simulink model "s_maglev_pid"  (R2021a)
settings: Solver=ode4  StartTime=0.0  StopTime=10.0  FixedStep=0.001  RelTol=1e-3
values from neighbouring files (symbols this model uses):
  g = 9.81    [config_maglev.m]
  IC_MAX = 3    [config_maglev.m]
  Kff_b = ic0 / xb0    [d_maglev_pi_piv.m]
  Ki_c = wn_c^2 * tau_c / Kc_dc    [d_maglev_pi_piv.m]
  Km = 6.5308e-5    (= 6.5308e-05)    [config_maglev.m]
  Kp_c = (2*zeta_c*wn_c*tau_c - 1) / Kc_dc    [d_maglev_pi_piv.m]
  Lc = 0.4125    [config_maglev.m]    (also in setup_maglev.m = 0.374)
  maglev_km = [xbfit; Km_xb_array]'    [load_variable_km.m]
  MAX_XB_WDUP = 1    [setup_maglev.m]
  Mb = 0.068    [config_maglev.m]
  Rc = 10    [config_maglev.m]    (also in setup_maglev.m)
  Tb = 0.014    [config_maglev.m]
  VMAX_AMP = 24    [config_maglev.m]
  xb0 = 6e-3    (= 0.006)    [setup_maglev.m]
  XB_REF_RATE = 5e-3    (= 0.005)    [setup_maglev.m]
undefined symbols (not defined in the file or in its folder): Ctuned, CtunedNom
libraries: pid_lib x2
settings Model: Creator=MLevis  LastModifiedBy=MLevis
settings DataIOCC: ReturnWorkspaceOutputs=off

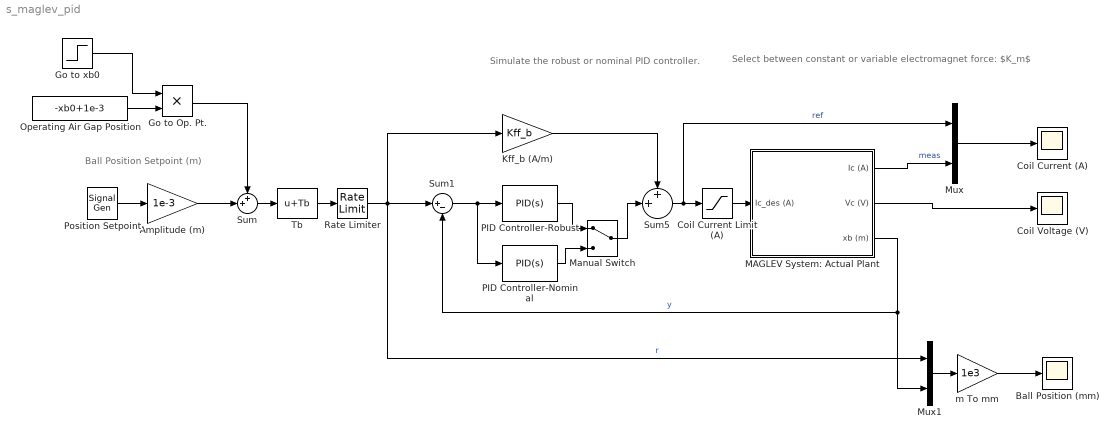
== system s_maglev_pid ==
  note: Simulate the robust or nominal PID controller.
  note: Select between constant or variable electromagnet force: $K_m$
  note: Ball Position Setpoint (m)
  Amplitude (m) : Gain  Gain=1e-3  SaturateOnIntegerOverflow=on  OutDataTypeStr=Inherit: Same as input  ParamDataTypeStr=Inherit: Same as input
  Ball Position (mm) : Scope
  Coil Current Limit (A) : Saturate  UpperLimit=IC_MAX  LowerLimit=0
  Coil Current (A) : Scope
  Coil Voltage (V) : Scope
  Go to Op. Pt. : Product  RndMeth=Zero
  Go to xb0 : Step  Time=2  SampleTime=0
  Kff_b (A/m) : Gain  Gain=Kff_b  SaturateOnIntegerOverflow=on  OutDataTypeStr=Inherit: Same as input  ParamDataTypeStr=Inherit: Same as input
  MAGLEV System: Actual Plant : Subsystem
  Manual Switch : ManualSwitch
  Mux : Mux  Inputs=2
  Mux1 : Mux  Inputs=2
  Operating Air Gap Position : Constant  Value=-xb0+1e-3
  PID Controller-Nominal : pid_lib/PID Controller  Controller=PID  Form=Parallel  TimeDomain=Continuous-time  UseExternalTs=off  SampleTime=-1  IntegratorMethod=Forward Euler  FilterMethod=Forward Euler  ControllerParametersSource=internal  P=CtunedNom.Kp  I=CtunedNom.Ki  D=CtunedNom.Kd  UseFilter=on  N=1/CtunedNom.Tf  TunerSelectOption=Transfer Function Based (PID Tuner App)  InitialConditionSource=internal  InitialConditionForIntegrator=0  InitialConditionForFilter=0  DifferentiatorICPrevScaledInput=0  ExternalReset=none  TrackingMode=off  Kt=1  LimitOutput=on  SatLimitsSource=internal  UpperSaturationLimit=MAX_XB_WDUP  LowerSaturationLimit=-MAX_XB_WDUP  LinearizeAsGain=on  AntiWindupMode=back-calculation  Kb=1  POutMin=[]  POutMax=[]  IOutMin=[]  IOutMax=[]  DOutMin=[]  DOutMax=[]  NOutMin=[]  NOutMax=[]  SumOutMin=[]  SumOutMax=[]  SaturationOutMin=[]  SaturationOutMax=[]  PParamMin=[]  PParamMax=[]  IParamMin=[]  IParamMax=[]  DParamMin=[]  DParamMax=[]  NParamMin=[]  NParamMax=[]  KbParamMin=[]  KbParamMax=[]  KtParamMin=[]  KtParamMax=[]  KbOutMin=[]  KbOutMax=[]  KtOutMin=[]  KtOutMax=[]  IntegratorOutMin=[]  IntegratorOutMax=[]  FilterOutMin=[]  FilterOutMax=[]  SumI1OutMin=[]  SumI1OutMax=[]  SumI2OutMin=[]  SumI2OutMax=[]  SumI3OutMin=[]  SumI3OutMax=[]  SumI4OutMin=[]  SumI4OutMax=[]  SumDOutMin=[]  SumDOutMax=[]  DifferentiatorOutMin=[]  DifferentiatorOutMax=[]  FilterDiffOutCoefMin=[]  FilterDiffOutCoefMax=[]  ReciprocalOutMin=[]  ReciprocalOutMax=[]  SumDenOutMin=[]  SumDenOutMax=[]  SumNumOutMin=[]  SumNumOutMax=[]  DivideOutMin=[]  DivideOutMax=[]  UdiffTsProdOutMin=[]  UdiffTsProdOutMax=[]  NTsProdOutMin=[]  NTsProdOutMax=[]  UintegralTsProdOutMin=[]  UintegralTsProdOutMax=[]  UngainTsProdOutMin=[]  UngainTsProdOutMax=[]  IntegratorContinuousStateAttributes=''  IntegratorStateMustResolveToSignalObject=off  IntegratorRTWStateStorageClass=Auto  FilterContinuousStateAttributes=''  FilterStateMustResolveToSignalObject=off  FilterRTWStateStorageClass=Auto  ParallelPVariant=InternalParameters  IdealPVariant=Disabled  IVariant=InternalParameters  DVariant=InternalParameters  IntegratorVariant=Continuous  SatVariant=Enabled  AWVariant=BackCalculation  PCopyVariant=Disabled  TRVariant=Disabled  FdbkBlocksVariant=Forward  IdealPFdbkVariant=Disabled  SatFdbkVariant=Disabled  DerivativeFilterVariant=ContFilter  NVariant=InternalParameters  NCopyVariant=Disabled  FilterICVariant=InternalICsFilter  IntegratorICVariant=InternalICs  ExternalResetVariant=Disabled  TRSumVariant=Passthrough  SumFdbkVariant=Disabled  SumVariant=Sum_PID  TsampFilterVariant=InternalTs  TsampNgainVariant=Passthrough  TsampIntegralVariant=Passthrough  ExternalSaturationOutDataTypeStr=Inherit: Same as second input
  PID Controller-Robust : pid_lib/PID Controller  Controller=PID  Form=Parallel  TimeDomain=Continuous-time  UseExternalTs=off  SampleTime=-1  IntegratorMethod=Forward Euler  FilterMethod=Forward Euler  ControllerParametersSource=internal  P=Ctuned.Kp  I=Ctuned.Ki  D=Ctuned.Kd  UseFilter=on  N=1/Ctuned.Tf  TunerSelectOption=Transfer Function Based (PID Tuner App)  InitialConditionSource=internal  InitialConditionForIntegrator=0  InitialConditionForFilter=0  DifferentiatorICPrevScaledInput=0  ExternalReset=none  TrackingMode=off  Kt=1  LimitOutput=on  SatLimitsSource=internal  UpperSaturationLimit=MAX_XB_WDUP  LowerSaturationLimit=-MAX_XB_WDUP  LinearizeAsGain=on  AntiWindupMode=back-calculation  Kb=1  POutMin=[]  POutMax=[]  IOutMin=[]  IOutMax=[]  DOutMin=[]  DOutMax=[]  NOutMin=[]  NOutMax=[]  SumOutMin=[]  SumOutMax=[]  SaturationOutMin=[]  SaturationOutMax=[]  PParamMin=[]  PParamMax=[]  IParamMin=[]  IParamMax=[]  DParamMin=[]  DParamMax=[]  NParamMin=[]  NParamMax=[]  KbParamMin=[]  KbParamMax=[]  KtParamMin=[]  KtParamMax=[]  KbOutMin=[]  KbOutMax=[]  KtOutMin=[]  KtOutMax=[]  IntegratorOutMin=[]  IntegratorOutMax=[]  FilterOutMin=[]  FilterOutMax=[]  SumI1OutMin=[]  SumI1OutMax=[]  SumI2OutMin=[]  SumI2OutMax=[]  SumI3OutMin=[]  SumI3OutMax=[]  SumI4OutMin=[]  SumI4OutMax=[]  SumDOutMin=[]  SumDOutMax=[]  DifferentiatorOutMin=[]  DifferentiatorOutMax=[]  FilterDiffOutCoefMin=[]  FilterDiffOutCoefMax=[]  ReciprocalOutMin=[]  ReciprocalOutMax=[]  SumDenOutMin=[]  SumDenOutMax=[]  SumNumOutMin=[]  SumNumOutMax=[]  DivideOutMin=[]  DivideOutMax=[]  UdiffTsProdOutMin=[]  UdiffTsProdOutMax=[]  NTsProdOutMin=[]  NTsProdOutMax=[]  UintegralTsProdOutMin=[]  UintegralTsProdOutMax=[]  UngainTsProdOutMin=[]  UngainTsProdOutMax=[]  IntegratorContinuousStateAttributes=''  IntegratorStateMustResolveToSignalObject=off  IntegratorRTWStateStorageClass=Auto  FilterContinuousStateAttributes=''  FilterStateMustResolveToSignalObject=off  FilterRTWStateStorageClass=Auto  ParallelPVariant=InternalParameters  IdealPVariant=Disabled  IVariant=InternalParameters  DVariant=InternalParameters  IntegratorVariant=Continuous  SatVariant=Enabled  AWVariant=BackCalculation  PCopyVariant=Disabled  TRVariant=Disabled  FdbkBlocksVariant=Forward  IdealPFdbkVariant=Disabled  SatFdbkVariant=Disabled  DerivativeFilterVariant=ContFilter  NVariant=InternalParameters  NCopyVariant=Disabled  FilterICVariant=InternalICsFilter  IntegratorICVariant=InternalICs  ExternalResetVariant=Disabled  TRSumVariant=Passthrough  SumFdbkVariant=Disabled  SumVariant=Sum_PID  TsampFilterVariant=InternalTs  TsampNgainVariant=Passthrough  TsampIntegralVariant=Passthrough  ExternalSaturationOutDataTypeStr=Inherit: Same as second input
  Position Setpoint : SignalGenerator  WaveForm=square  Frequency=.25
  Rate Limiter : RateLimiter  RisingSlewLimit=XB_REF_RATE  FallingSlewLimit=-XB_REF_RATE  SampleTimeMode=inherited
  Sum : Sum  Inputs=++|
  Sum1 : Sum  Inputs=|+-
  Sum5 : Sum  Inputs=++|  InputSameDT=on  SaturateOnIntegerOverflow=on  OutDataTypeStr=Inherit: Same as first input
  Tb : Bias  Bias=Tb
  m To mm : Gain  Gain=1e3  SaturateOnIntegerOverflow=on  OutDataTypeStr=Inherit: Same as input  ParamDataTypeStr=Inherit: Same as input
  wires:
  Go to Op. Pt./1 -> Sum/1
  Coil Current Limit (A)/1 -> MAGLEV System: Actual Plant/1(Ic_des (A))
  Amplitude (m)/1 -> Sum/2
  Mux1/1 -> m To mm/1
  MAGLEV System: Actual Plant/2(Vc (V)) -> Coil Voltage (V)/1
  m To mm/1 -> Ball Position (mm)/1
  Operating Air Gap Position/1 -> Go to Op. Pt./2
  Position Setpoint/1 -> Amplitude (m)/1
  MAGLEV System: Actual Plant/3(xb (m)) -> Mux1/2, Sum1/2  "y"
  Sum/1 -> Tb/1
  MAGLEV System: Actual Plant/1(Ic (A)) -> Mux/2  "meas"
  Mux/1 -> Coil Current (A)/1
  Tb/1 -> Rate Limiter/1
  Go to xb0/1 -> Go to Op. Pt./1
  Rate Limiter/1 -> Mux1/1, Sum1/1, Kff_b (A/m)/1  "r"
  Kff_b (A/m)/1 -> Sum5/1
  Sum5/1 -> Mux/1, Coil Current Limit (A)/1  "ref"
  Sum1/1 -> PID Controller-Nominal/1, PID Controller-Robust/1
  PID Controller-Robust/1 -> Manual Switch/1
  PID Controller-Nominal/1 -> Manual Switch/2
  Manual Switch/1 -> Sum5/2

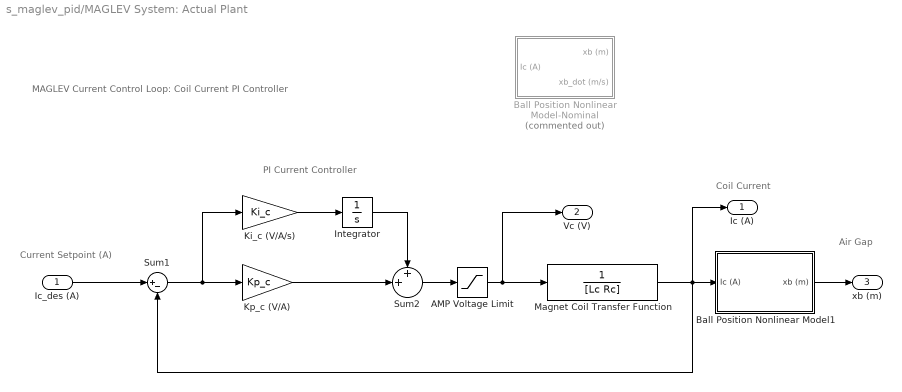
== system s_maglev_pid/MAGLEV System: Actual Plant ==
  note: Coil Current
  note: Air Gap
  note: MAGLEV Current Control Loop:
      | Coil Current PI Controller
  note: Current Setpoint (A)
  note: PI Current Controller
  Ic_des (A) : Inport
  AMP Voltage Limit : Saturate  UpperLimit=VMAX_AMP  LowerLimit=-VMAX_AMP
  Ball Position Nonlinear Model-Nominal : Subsystem  Commented=on
  Ball Position Nonlinear Model1 : Subsystem
  Integrator : Integrator  LimitOutput=on  UpperSaturationLimit=VMAX_AMP  LowerSaturationLimit=-VMAX_AMP
  Ki_c (V/A/s) : Gain  Gain=Ki_c  SaturateOnIntegerOverflow=on  OutDataTypeStr=Inherit: Same as input  ParamDataTypeStr=Inherit: Same as input
  Kp_c (V/A) : Gain  Gain=Kp_c  SaturateOnIntegerOverflow=on  OutDataTypeStr=Inherit: Same as input  ParamDataTypeStr=Inherit: Same as input
  Magnet Coil Transfer Function : TransferFcn  Denominator=[Lc Rc]
  Sum1 : Sum  Inputs=|+-
  Sum2 : Sum  Inputs=++|  InputSameDT=on  SaturateOnIntegerOverflow=on  OutDataTypeStr=Inherit: Same as first input
  Ic (A) : Outport  InitialOutput=0
  Vc (V) : Outport  Port=2  InitialOutput=0
  xb (m) : Outport  Port=3  InitialOutput=0
  wires:
  AMP Voltage Limit/1 -> Vc (V)/1, Magnet Coil Transfer Function/1
  Ki_c (V/A/s)/1 -> Integrator/1
  Integrator/1 -> Sum2/1
  Sum2/1 -> AMP Voltage Limit/1
  Kp_c (V/A)/1 -> Sum2/2
  Magnet Coil Transfer Function/1 -> Ball Position Nonlinear Model1/1(Ic (A)), Sum1/2, Ic (A)/1
  Sum1/1 -> Ki_c (V/A/s)/1, Kp_c (V/A)/1
  Ic_des (A)/1 -> Sum1/1
  Ball Position Nonlinear Model1/1(xb (m)) -> xb (m)/1

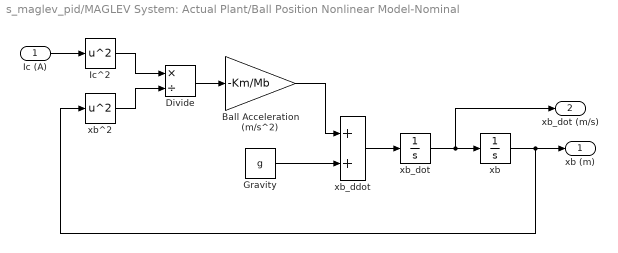
== system s_maglev_pid/MAGLEV System: Actual Plant/Ball Position Nonlinear Model-Nominal ==
  Ic (A) : Inport
  Ball Acceleration (m/s^2) : Gain  Gain=-Km/Mb
  Divide : Product  Inputs=*/
  Gravity : Constant  Value=g
  Ic^2 : Math  Operator=square  SignedPower=on  SaturateOnIntegerOverflow=on
  xb : Integrator  InitialCondition=Tb  LimitOutput=on  UpperSaturationLimit=Tb  LowerSaturationLimit=0
  xb^2 : Math  Operator=square  SignedPower=on  SaturateOnIntegerOverflow=on
  xb_ddot : Sum
  xb_dot : Integrator
  xb (m) : Outport
  xb_dot (m/s) : Outport  Port=2
  wires:
  xb^2/1 -> Divide/2
  Ic (A)/1 -> Ic^2/1
  Divide/1 -> Ball Acceleration (m/s^2)/1
  Ic^2/1 -> Divide/1
  Ball Acceleration (m/s^2)/1 -> xb_ddot/1
  Gravity/1 -> xb_ddot/2
  xb_ddot/1 -> xb_dot/1
  xb_dot/1 -> xb/1, xb_dot (m/s)/1
  xb/1 -> xb (m)/1, xb^2/1

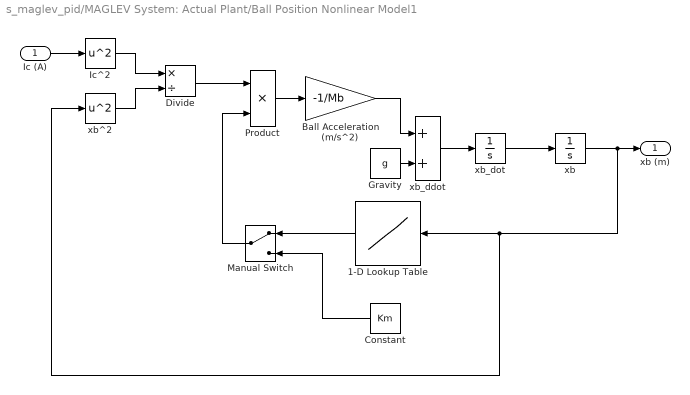
== system s_maglev_pid/MAGLEV System: Actual Plant/Ball Position Nonlinear Model1 ==
  Ic (A) : Inport
  1-D Lookup Table : Lookup_n-D  NumberOfTableDimensions=1  LookupTableObject=maglev_km  BreakpointsForDimension1=maglev_km(:,1)  IndexSearchMethod=Linear search  Table=maglev_km(:,2)  InternalRulePriority=Speed  RndMeth=Simplest  InputSameDT=on
  Ball Acceleration (m/s^2) : Gain  Gain=-1/Mb
  Constant : Constant  Value=Km
  Divide : Product  Inputs=*/
  Gravity : Constant  Value=g
  Ic^2 : Math  Operator=square  SignedPower=on  SaturateOnIntegerOverflow=on
  Manual Switch : ManualSwitch
  Product : Product
  xb : Integrator  InitialCondition=Tb  LimitOutput=on  UpperSaturationLimit=Tb  LowerSaturationLimit=0
  xb^2 : Math  Operator=square  SignedPower=on  SaturateOnIntegerOverflow=on
  xb_ddot : Sum
  xb_dot : Integrator
  xb (m) : Outport
  wires:
  Constant/1 -> Manual Switch/2
  Manual Switch/1 -> Product/2
  1-D Lookup Table/1 -> Manual Switch/1
  Product/1 -> Ball Acceleration (m/s^2)/1
  Divide/1 -> Product/1
  xb/1 -> xb (m)/1, 1-D Lookup Table/1, xb^2/1
  xb_dot/1 -> xb/1
  xb_ddot/1 -> xb_dot/1
  Gravity/1 -> xb_ddot/2
  Ball Acceleration (m/s^2)/1 -> xb_ddot/1
  Ic^2/1 -> Divide/1
  Ic (A)/1 -> Ic^2/1
  xb^2/1 -> Divide/2
